simulink model "smib"  (R2021b)
settings: Solver=VariableStepAuto  StartTime=0.0  StopTime=10  MaxStep=0.1  RelTol=1e-3
settings Model: Creator=wei  LastModifiedBy=wei

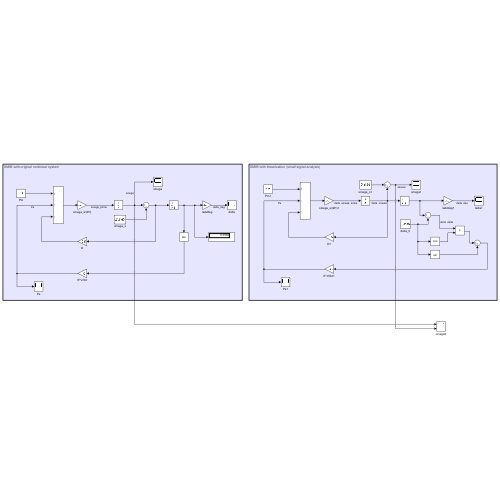
[thumbnail: Simulink's stored preview of the top-level diagram]
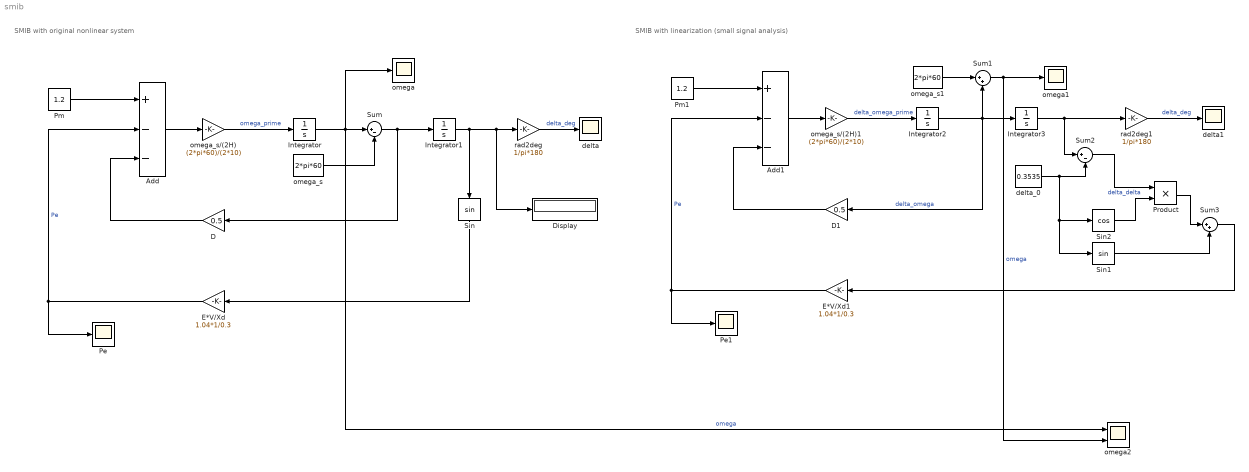
== system smib ==
  note: SMIB with original nonlinear system
  note: SMIB with linearization (small signal analysis)
  Add : Sum  Inputs=+--
  Add1 : Sum  Inputs=+--
  D : Gain  Gain=0.5
  D1 : Gain  Gain=0.5
  Display : Display
  E*V/Xd : Gain  Gain=1.04*1/0.3
  E*V/Xd1 : Gain  Gain=1.04*1/0.3
  Integrator : Integrator
  Integrator1 : Integrator  LimitOutput=on  UpperSaturationLimit=2*pi  LowerSaturationLimit=0
  Integrator2 : Integrator
  Integrator3 : Integrator  LimitOutput=on  UpperSaturationLimit=2*pi  LowerSaturationLimit=0
  Pe : Scope
  Pe1 : Scope
  Pm : Constant  Value=1.2
  Pm1 : Constant  Value=1.2
  Product : Product
  Sin : Trigonometry
  Sin1 : Trigonometry
  Sin2 : Trigonometry  Operator=cos
  Sum : Sum  Inputs=|+-
  Sum1 : Sum  Inputs=|++
  Sum2 : Sum  Inputs=|+-
  Sum3 : Sum  Inputs=|++
  delta : Scope
  delta1 : Scope
  delta_0 : Constant  Value=0.3535
  omega : Scope
  omega1 : Scope
  omega2 : Scope  NumInputPorts=2
  omega_s : Constant  Value=2*pi*60
  omega_s/(2H) : Gain  Gain=(2*pi*60)/(2*10)
  omega_s/(2H)1 : Gain  Gain=(2*pi*60)/(2*10)
  omega_s1 : Constant  Value=2*pi*60
  rad2deg : Gain  Gain=1/pi*180
  rad2deg1 : Gain  Gain=1/pi*180
  wires:
  omega_s/1 -> Sum/2
  Integrator/1 -> omega2/1, Sum/1, omega/1  "omega"
  Sum/1 -> D/1, Integrator1/1
  Pm/1 -> Add/1
  D/1 -> Add/3
  E*V/Xd/1 -> Add/2, Pe/1  "Pe"
  Sin/1 -> E*V/Xd/1
  Add/1 -> omega_s/(2H)/1
  omega_s/(2H)/1 -> Integrator/1  "omega_prime"
  omega_s/(2H)1/1 -> Integrator2/1  "delta_omega_prime"
  E*V/Xd1/1 -> Add1/2, Pe1/1  "Pe"
  Add1/1 -> omega_s/(2H)1/1
  D1/1 -> Add1/3
  Integrator2/1 -> Integrator3/1, D1/1, Sum1/2  "delta_omega"
  Integrator3/1 -> Sum2/1, rad2deg1/1
  Pm1/1 -> Add1/1
  Integrator1/1 -> Display/1, rad2deg/1, Sin/1
  rad2deg/1 -> delta/1  "delta_deg"
  rad2deg1/1 -> delta1/1  "delta_deg"
  omega_s1/1 -> Sum1/1
  Sum1/1 -> omega2/2, omega1/1  "omega"
  delta_0/1 -> Sin2/1, Sin1/1, Sum2/2
  Sum2/1 -> Product/1  "delta_delta"
  Sin2/1 -> Product/2
  Sin1/1 -> Sum3/2
  Product/1 -> Sum3/1
  Sum3/1 -> E*V/Xd1/1
